simulink model "OfflineSim_V6_nobow"  (R2015a)
settings: Solver=ode3  SolverMode=SingleTasking  StartTime=0.0  StopTime=inf  FixedStep=0.01  RelTol=1e-3
undefined symbols (not defined in the file): BiasOffset, eta_dot_ini, K2, L1, L2, L3
libraries: sldrtlib x1, simulink x1
settings Model: CovMetricSettings=dwe  CovHtmlReporting=off  covSaveCumulativeToWorkspaceVar=off  CovSaveSingleToWorkspaceVar=off  CovExternalEMLEnable=on  Creator=ssp  LastModifiedBy=ssp
settings DataIOCC: LimitDataPoints=off  SaveFormat=Dataset
settings DebuggingCC: SFUnexpectedBacktrackingDiag=error  SFNoUnconditionalDefaultTransitionDiag=error
settings HardwareCC: ProdBitPerPointer=64  ProdLargestAtomicFloat=Float  ProdIntDivRoundTo=Zero  ProdEndianess=LittleEndian  ProdHWDeviceType=Specified
settings ModelReferenceCC: PropagateSignalLabelsOutOfModel=on
settings GRTTargetCC: TargetLangStandard=C99 (ISO)  GeneratePreprocessorConditionals=Use local settings

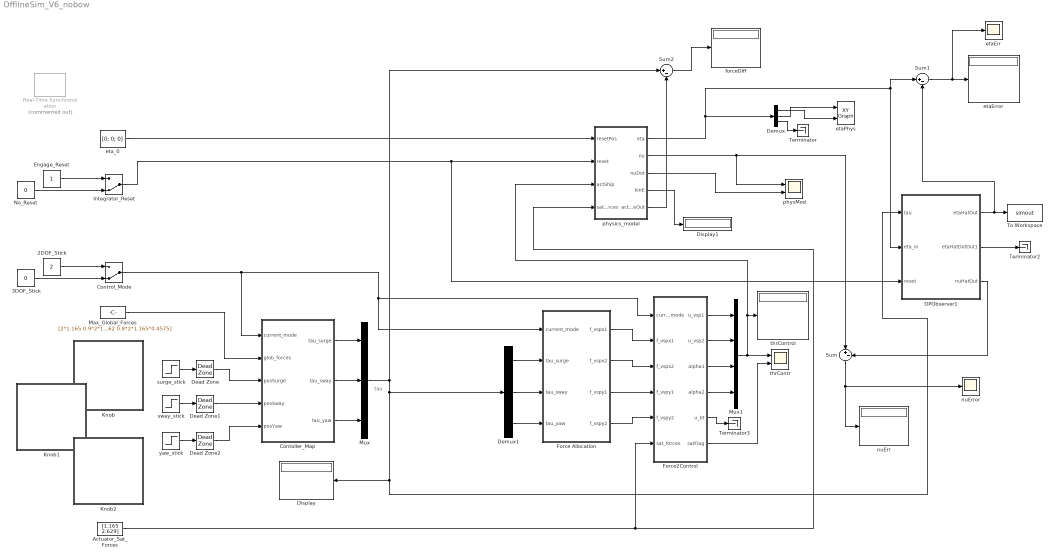
== system OfflineSim_V6_nobow ==
  note: tau
  2DOF_Stick : Constant  Value=2
  3DOF_Stick : Constant  Value=0
  Actuator_Sat_Forces : Constant  Value=[1.165 2.629]
  Contoller_Map : MATLAB Function  TreatAsAtomicUnit=on
      settings: PermitHierarchicalResolution=ParametersOnly
  Control_Mode : ManualSwitch  CurrentSetting=0
  DPObserver1 : Subsystem
  Dead Zone : DeadZone  LowerValue=-0.05  UpperValue=0.05  SaturateOnIntegerOverflow=on
  Dead Zone1 : DeadZone  LowerValue=-0.05  UpperValue=0.05  SaturateOnIntegerOverflow=on
  Dead Zone2 : DeadZone  LowerValue=-0.05  UpperValue=0.05  SaturateOnIntegerOverflow=on
  Demux : Demux  Outputs=3
  Demux1 : Demux  Outputs=3
  Display : Display
  Display1 : Display
  Engage_Reset : Constant
  Force Allocation : MATLAB Function  TreatAsAtomicUnit=on
      settings: PermitHierarchicalResolution=ParametersOnly
  Force2Control : MATLAB Function  TreatAsAtomicUnit=on
      settings: PermitHierarchicalResolution=ParametersOnly
  Integrator_Reset : ManualSwitch  CurrentSetting=0
  Knob : Subsystem  DialogController=hmiCreateDDGDialog  IsWebBlock=on  mask(MathWorksWebBlock){webBlockId=4a71b7a3-6536-403a-8bad-6aeba5635746, webBlockType=continuousknob, ShowInLibBrowser=on, ShowInitialText=on, HMISrcModelName=OfflineSim_V6_nobow}
      mask prompts: webBlockId "WebBlock Id"; webBlockType "WebBlock Type"; HMISrcModelName "Source Model"
      mask help: SimulinkHMI:dialogs:ContinuousKnobDialogDesc
      mask Help: helpview([docroot '/mapfiles/simulink.map'], 'hmi_knob')
      mask Display:
      | if strcmp(get_param(bdroot(gcb),'BlockDiagramType'), 'library')
      |     image([(matlabroot) '/toolbox/simulink/hmi/icons/ContinuousKnob.png']);
      | end
  Knob1 : Subsystem  DialogController=hmiCreateDDGDialog  IsWebBlock=on  mask(MathWorksWebBlock){webBlockId=6469085c-47a6-49a2-9ebc-fb6a8e18618c, webBlockType=continuousknob, ShowInLibBrowser=on, ShowInitialText=on, HMISrcModelName=OfflineSim_V6_nobow}
      mask prompts: webBlockId "WebBlock Id"; webBlockType "WebBlock Type"; HMISrcModelName "Source Model"
      mask help: SimulinkHMI:dialogs:ContinuousKnobDialogDesc
      mask Help: helpview([docroot '/mapfiles/simulink.map'], 'hmi_knob')
      mask Display:
      | if strcmp(get_param(bdroot(gcb),'BlockDiagramType'), 'library')
      |     image([(matlabroot) '/toolbox/simulink/hmi/icons/ContinuousKnob.png']);
      | end
  Knob2 : Subsystem  DialogController=hmiCreateDDGDialog  IsWebBlock=on  mask(MathWorksWebBlock){webBlockId=01ffebd2-c22d-44d7-8fc7-1049d6cabe31, webBlockType=continuousknob, ShowInLibBrowser=on, ShowInitialText=on, HMISrcModelName=OfflineSim_V6_nobow}
      mask prompts: webBlockId "WebBlock Id"; webBlockType "WebBlock Type"; HMISrcModelName "Source Model"
      mask help: SimulinkHMI:dialogs:ContinuousKnobDialogDesc
      mask Help: helpview([docroot '/mapfiles/simulink.map'], 'hmi_knob')
      mask Display:
      | if strcmp(get_param(bdroot(gcb),'BlockDiagramType'), 'library')
      |     image([(matlabroot) '/toolbox/simulink/hmi/icons/ContinuousKnob.png']);
      | end
  Max_Global_Forces : Constant  Value=[2*1.165 0.9*2*1.165*sin(atan(0.062/0.4575)) 0.95*2*1.165*0.062 0.8*2*1.165*0.4575]
  Mux : Mux  Inputs=3
  Mux1 : Mux
  No_Reset : Constant  Value=0
  Real-Time Synchronization : sldrtlib/Real-Time Synchronization  Commented=on  SampleTime=0.1  MaxMissedTicks=10  ShowMissedTicks=off  YieldWhenWaiting=off
  Sum : Sum  Inputs=|+-
  Sum1 : Sum  Inputs=|+-
  Sum2 : Sum  Inputs=|+-
  Terminator : Terminator
  Terminator2 : Terminator
  Terminator3 : Terminator
  To Workspace : ToWorkspace  VariableName=simout  SampleTime=-1
  etaErr : Scope
      settings: TimeRange=50  ShowLegends=on  MaxDataPoints=5000  SaveToWorkspace=off  SaveName=ScopeData2  YMin=-1.00000  YMax=1.00000  SampleTime=-1
  etaError : Display
  etaPhys : simulink/Sinks/XY Graph  xmin=-10  xmax=10  ymin=-10  ymax=10  st=-1
  eta_0 : Constant  Value=[0; 0; 0]
  forceDiff : Display
  nuErr : Display
  nuError : Scope
      settings: TimeRange=50  ShowLegends=on  MaxDataPoints=5000  SaveToWorkspace=off  YMin=-1.00000  YMax=1.00000  SampleTime=-1
  physMod : Scope  NumInputPorts=2
      settings: TimeRange=50  ShowLegends=on  MaxDataPoints=5000  SaveToWorkspace=off  SaveName=ScopeData  YMin=-0.00713~-5  YMax=0.05351~5  SampleTime=-1
  physics_model : Subsystem
  surge_stick : Step  Time=0  After=0  SampleTime=0.01
  sway_stick : Step  Time=0  After=0  SampleTime=0
  thrContr : Scope  NumInputPorts=2
      settings: TimeRange=50  ShowLegends=on  MaxDataPoints=5000  SaveToWorkspace=off  YMin=-0.3927~-5  YMax=3.53429~5  SampleTime=-1
  thrControl : Display
  yaw_stick : Step  Time=0  After=0  SampleTime=0
  wires:
  Engage_Reset/1 -> Integrator_Reset/1
  No_Reset/1 -> Integrator_Reset/2
  Contoller_Map/1(tau_surge) -> Mux/1
  Contoller_Map/2(tau_sway) -> Mux/2
  Contoller_Map/3(tau_yaw) -> Mux/3
  Max_Global_Forces/1 -> Contoller_Map/2(glob_forces)
  2DOF_Stick/1 -> Control_Mode/1
  3DOF_Stick/1 -> Control_Mode/2
  Control_Mode/1 -> Contoller_Map/1(current_mode), Force2Control/1(current_mode), Force Allocation/1(current_mode)
  surge_stick/1 -> Dead Zone/1
  sway_stick/1 -> Dead Zone1/1
  yaw_stick/1 -> Dead Zone2/1
  eta_0/1 -> physics_model/1(resetPos)
  Integrator_Reset/1 -> DPObserver1/3("reset "), physics_model/2(reset)
  Mux/1 -> Sum2/1, Display/1, DPObserver1/1(tau), Demux1/1
  physics_model/1(eta) -> Demux/1, DPObserver1/2(eta_in), Sum1/1
  physics_model/2(nu) -> physMod/1, Sum/1
  Demux/1 -> etaPhys/2
  Demux/2 -> etaPhys/1
  Demux/3 -> Terminator/1
  physics_model/3(nuDot) -> physMod/2
  physics_model/4(kinE) -> Display1/1
  Demux1/1 -> Force Allocation/2(tau_surge)
  Demux1/2 -> Force Allocation/3(tau_sway)
  Demux1/3 -> Force Allocation/4(tau_yaw)
  Force Allocation/1(f_vspx1) -> Force2Control/2(f_vspx1)
  Force Allocation/2(f_vspx2) -> Force2Control/3(f_vspx2)
  Mux1/1 -> thrContr/1, physics_model/3(actShip), thrControl/1
  Force2Control/1(u_vsp1) -> Mux1/1
  Force2Control/2(u_vsp2) -> Mux1/2
  Force2Control/6(satFlag) -> thrContr/2
  Actuator_Sat_Forces/1 -> physics_model/4(satForces), Force2Control/6(sat_forces)
  Dead Zone/1 -> Contoller_Map/3(posSurge)
  Dead Zone1/1 -> Contoller_Map/4(posSway)
  Dead Zone2/1 -> Contoller_Map/5(posYaw)
  DPObserver1/2(etaHatDotOut1) -> Terminator2/1
  DPObserver1/3(nuHatOut) -> Sum/2
  Sum/1 -> nuError/1, nuErr/1
  DPObserver1/1(etaHatOut) -> Sum1/2, To Workspace/1
  Sum1/1 -> etaErr/1, etaError/1
  Force Allocation/3(f_vspy1) -> Force2Control/4(f_vspy1)
  Force Allocation/4(f_vspy2) -> Force2Control/5(f_vspy2)
  Force2Control/5(u_bt) -> Terminator3/1
  Force2Control/3(alpha1) -> Mux1/3
  Force2Control/4(alpha2) -> Mux1/4
  physics_model/5(actForceOut) -> Sum2/2
  Sum2/1 -> forceDiff/1

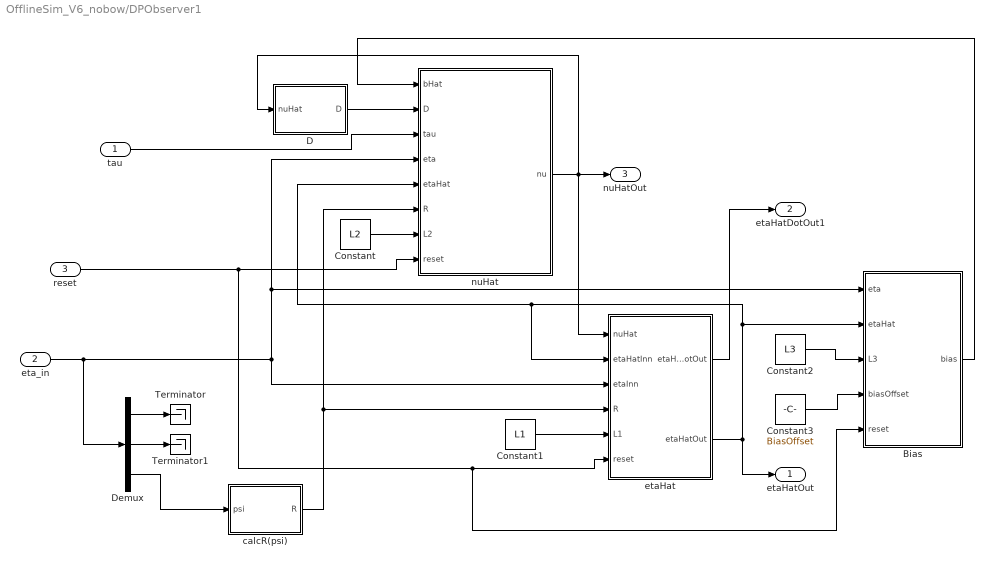
== system OfflineSim_V6_nobow/DPObserver1 ==
  tau : Inport
  eta_in : Inport  Port=2
  "reset " : Inport  Port=3
  Bias : Subsystem
  Constant : Constant  Value=L2
  Constant1 : Constant  Value=L1
  Constant2 : Constant  Value=L3
  Constant3 : Constant  Value=BiasOffset
  D : MATLAB Function  TreatAsAtomicUnit=on
      settings: PermitHierarchicalResolution=ParametersOnly
  Demux : Demux  Outputs=3
  Terminator : Terminator
  Terminator1 : Terminator
  "calcR(psi) " : MATLAB Function  TreatAsAtomicUnit=on
      settings: PermitHierarchicalResolution=ParametersOnly
  etaHat : Subsystem
  nuHat : Subsystem
  etaHatOut : Outport
  etaHatDotOut1 : Outport  Port=2
  nuHatOut : Outport  Port=3
  wires:
  "calcR(psi) "/1(R) -> nuHat/6(R), etaHat/4(R)
  etaHat/2(etaHatOut) -> etaHatOut/1, nuHat/5(etaHat), etaHat/2(etaHatInn), Bias/2(etaHat)
  tau/1 -> nuHat/3(tau)
  etaHat/1(etaHatDotOut) -> etaHatDotOut1/1
  nuHat/1(nu) -> etaHat/1(nuHat), D/1(nuHat), nuHatOut/1
  eta_in/1 -> Demux/1, nuHat/4(eta), Bias/1(eta), etaHat/3(etaInn)
  D/1(D) -> nuHat/2(D)
  Bias/1(bias) -> nuHat/1(bHat)
  Demux/3 -> "calcR(psi) "/1(psi)
  Constant/1 -> nuHat/7(L2)
  Constant2/1 -> Bias/3(L3)
  Constant3/1 -> Bias/4(biasOffset)
  Demux/1 -> Terminator/1
  Demux/2 -> Terminator1/1
  Constant1/1 -> etaHat/5(L1)
  "reset "/1 -> Bias/5(reset), etaHat/6(reset), nuHat/8(reset)

== system OfflineSim_V6_nobow/Knob ==

== system OfflineSim_V6_nobow/Knob1 ==

== system OfflineSim_V6_nobow/Knob2 ==

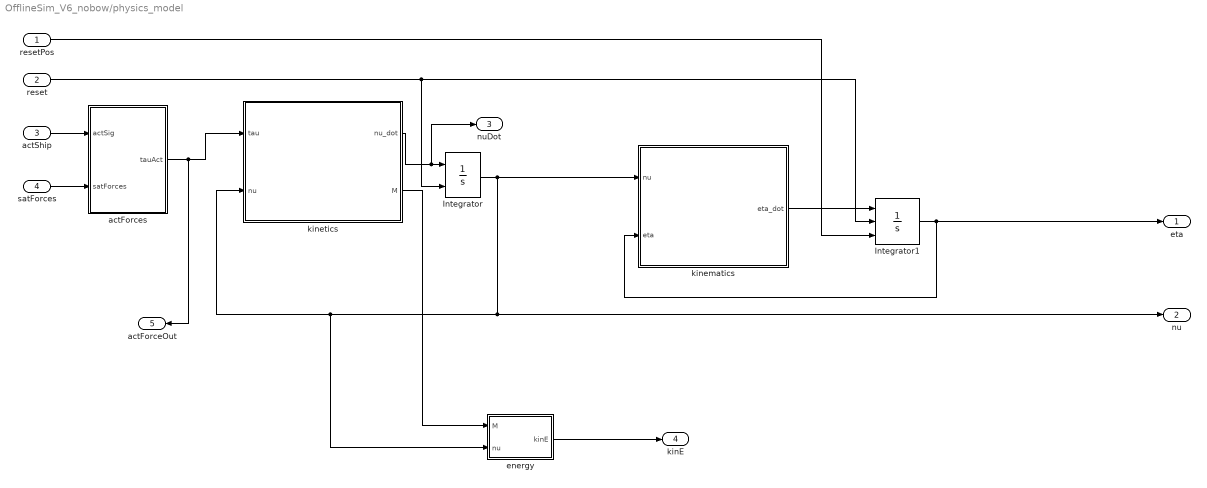
== system OfflineSim_V6_nobow/physics_model ==
  resetPos : Inport
  reset : Inport  Port=2
  actShip : Inport  Port=3
  satForces : Inport  Port=4
  Integrator : Integrator  ExternalReset=rising  InitialCondition=[0 0 0]'
  Integrator1 : Integrator  ExternalReset=rising  InitialConditionSource=external  InitialCondition=[0 0 0]'
  actForces : MATLAB Function  TreatAsAtomicUnit=on
      settings: PermitHierarchicalResolution=ParametersOnly
  energy : MATLAB Function  TreatAsAtomicUnit=on
      settings: PermitHierarchicalResolution=ParametersOnly
  kinematics : MATLAB Function  TreatAsAtomicUnit=on
      settings: PermitHierarchicalResolution=ParametersOnly
  kinetics : MATLAB Function  TreatAsAtomicUnit=on
      settings: PermitHierarchicalResolution=ParametersOnly
  eta : Outport
  nu : Outport  Port=2
  nuDot : Outport  Port=3
  kinE : Outport  Port=4
  actForceOut : Outport  Port=5
  wires:
  kinetics/1(nu_dot) -> nuDot/1, Integrator/1
  Integrator/1 -> nu/1, energy/2(nu), kinetics/2(nu), kinematics/1(nu)
  kinematics/1(eta_dot) -> Integrator1/1
  Integrator1/1 -> eta/1, kinematics/2(eta)
  reset/1 -> Integrator1/2, Integrator/2
  resetPos/1 -> Integrator1/3
  kinetics/2(M) -> energy/1(M)
  energy/1(kinE) -> kinE/1
  actShip/1 -> actForces/1(actSig)
  satForces/1 -> actForces/2(satForces)
  actForces/1(tauAct) -> actForceOut/1, kinetics/1(tau)

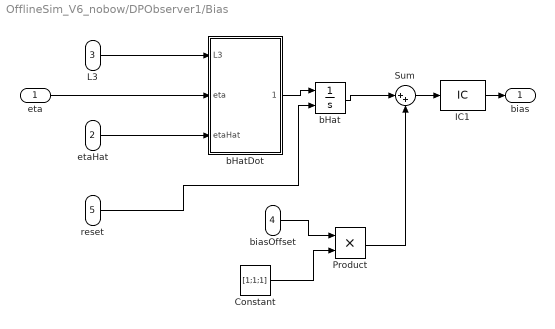
== system OfflineSim_V6_nobow/DPObserver1/Bias ==
  eta : Inport
  etaHat : Inport  Port=2
  L3 : Inport  Port=3
  biasOffset : Inport  Port=4  PortDimensions=1
  reset : Inport  Port=5
  Constant : Constant  Value=[1;1;1]
  IC1 : InitialCondition  Value=[0;0;0]
  Product : Product
  Sum : Sum  Inputs=|++
  bHat : Integrator  ExternalReset=rising
  bHatDot : MATLAB Function  TreatAsAtomicUnit=on
      settings: PermitHierarchicalResolution=ParametersOnly
  bias : Outport
  wires:
  bHatDot/1(bHatDot) -> bHat/1
  eta/1 -> bHatDot/2(eta)
  etaHat/1 -> bHatDot/3(etaHat)
  L3/1 -> bHatDot/1(L3)
  IC1/1 -> bias/1
  Sum/1 -> IC1/1
  biasOffset/1 -> Product/1
  Product/1 -> Sum/2
  Constant/1 -> Product/2
  bHat/1 -> Sum/1
  reset/1 -> bHat/2

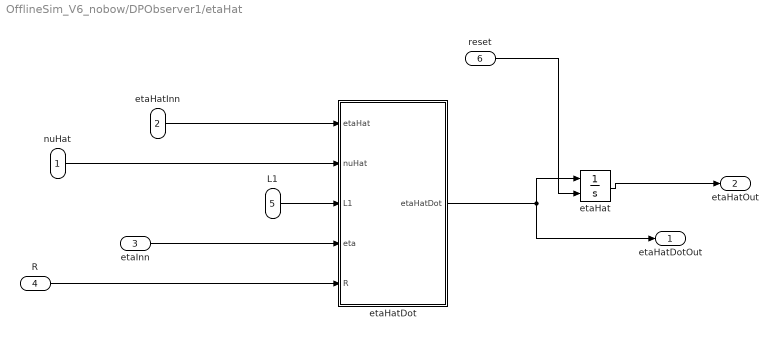
== system OfflineSim_V6_nobow/DPObserver1/etaHat ==
  nuHat : Inport
  etaHatInn : Inport  Port=2
  etaInn : Inport  Port=3
  R : Inport  Port=4
  L1 : Inport  Port=5
  reset : Inport  Port=6
  etaHat : Integrator  ExternalReset=rising  InitialCondition=eta_dot_ini
  etaHatDot : MATLAB Function  TreatAsAtomicUnit=on
      settings: PermitHierarchicalResolution=ParametersOnly
  etaHatDotOut : Outport
  etaHatOut : Outport  Port=2
  wires:
  etaHat/1 -> etaHatOut/1
  etaHatDot/1(etaHatDot) -> etaHat/1, etaHatDotOut/1
  L1/1 -> etaHatDot/3(L1)
  R/1 -> etaHatDot/5(R)
  nuHat/1 -> etaHatDot/2(nuHat)
  etaInn/1 -> etaHatDot/4(eta)
  etaHatInn/1 -> etaHatDot/1(etaHat)
  reset/1 -> etaHat/2

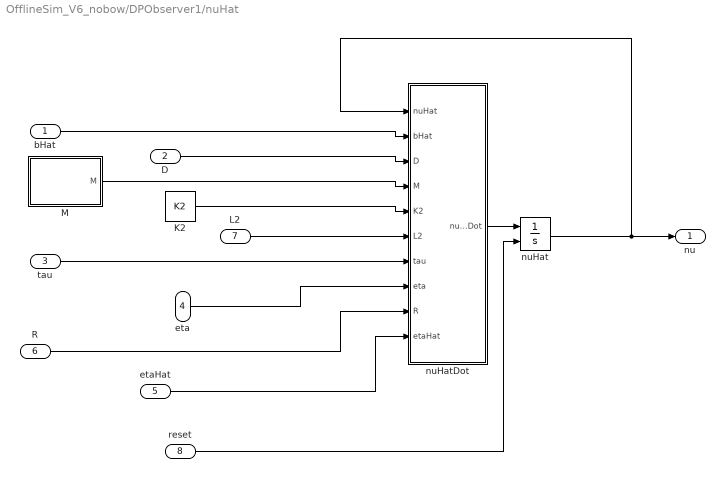
== system OfflineSim_V6_nobow/DPObserver1/nuHat ==
  bHat : Inport
  D : Inport  Port=2
  tau : Inport  Port=3
  eta : Inport  Port=4
  etaHat : Inport  Port=5
  R : Inport  Port=6
  L2 : Inport  Port=7
  reset : Inport  Port=8
  K2 : Constant  Value=K2
  M : MATLAB Function  TreatAsAtomicUnit=on
      settings: PermitHierarchicalResolution=ParametersOnly
  nuHat : Integrator  ExternalReset=rising  InitialCondition=[0;0;0]
  nuHatDot : MATLAB Function  TreatAsAtomicUnit=on
      settings: PermitHierarchicalResolution=ParametersOnly
  nu : Outport
  wires:
  K2/1 -> nuHatDot/5(K2)
  tau/1 -> nuHatDot/7(tau)
  bHat/1 -> nuHatDot/2(bHat)
  M/1(M) -> nuHatDot/4(M)
  nuHat/1 -> nuHatDot/1(nuHat), nu/1
  etaHat/1 -> nuHatDot/10(etaHat)
  R/1 -> nuHatDot/9(R)
  eta/1 -> nuHatDot/8(eta)
  nuHatDot/1(nuHatDot) -> nuHat/1
  D/1 -> nuHatDot/3(D)
  L2/1 -> nuHatDot/6(L2)
  reset/1 -> nuHat/2

== matlab function OfflineSim_V6_nobow/physics_model/kinematics ==
  data: nu input; eta_dot output; eta input
function eta_dot = CSE1_eta_dot(nu,eta)

psi = eta(3);

J = [cos(psi) -sin(psi) 0
     sin(psi) cos(psi)  0
     0        0         1];

eta_dot = J*nu;

== matlab function OfflineSim_V6_nobow/physics_model/kinetics ==
  data: tau input; nu_dot output; nu input; M output
function [nu_dot,M] = CSE1_nu_dot_corr(tau,nu)

u   = nu(1);
v   = nu(2);
r   = nu(3);

tau = [tau(1);tau(2);tau(3)];
%% MATRICES

m    = 14.79;   I_z  =  1.7600;   x_g = 0.0375;       % x_g  =  0.0460; % Table B.1


%% Added mass
X_ud  =     -2.0;											% Table B.1
Y_vd =     -10.0;	
N_vd =    -0.0;                                             % Table B.1 guestimate
Y_rd =      -0.0;	
N_rd =    -1.0;                                             % Table B.1

%% Total mass matrix
m_11 = m-X_ud;
m_22 = m-Y_vd;
m_23 = m*x_g-Y_rd;
m_32 = m*x_g-N_vd;
m_33 = I_z-N_rd;

M    = [m_11 0    0
        0    m_22 m_23
        0    m_32 m_33];
	
%% Damping coefficients
% Comments at the end of the lines indicate the old values used.
X_u		= -0.6555;		X_v		= 0;
X_uu 	= 0.3545;		X_vv	= -2.443;
X_uuu 	= -3.787;		X_vvv	= 0;

Y_v		= -1.33; 			Y_r		= -7.250; % Y_r
Y_vv	= -2.776;			Y_rr	= -3.450; % Y_rr
Y_vvv	= -64.91;			Y_rrr	= 0;
						
Y_rv	= -0.805;			Y_vr	= -0.845; % Y_rv, Y_vr

N_v		= 0;				N_r		= -1.900; % N_r
N_vv	= -0.2088;			N_rr	= -0.750; % N_rr
N_vvv	= 0;				N_rrr	= 0;
N_rv	= 0.130;			N_vr	= 0.080; % N_rv, N_vr

%% Correolis matrix

%from ItsLearning
%  c_13 = -(m-Y_vd)*v-(m*x_g-Y_rd)*r;
%  c_23 = (m-X_ud)*u;
% C    = [0     0     c_13
%         0     0     c_23
%         -c_13 -c_23 0   ];

%From Handbook of Marine Craft Hydr 1st ed pp.120
a1 = X_ud*u;
a2 = Y_vd*v-m*x_g;
C    = [0     0     a2
        0     0    -a1
       -a2    a1    0   ];

%% Assembly of the damping matrix
d_11 = -X_u - X_uu*abs(u) - X_uuu*u^2;
d_22 = -Y_v - Y_vv*abs(v) - Y_vvv*v^2 - Y_rv*abs(r);
d_33 = -N_r - N_rr*abs(r) - N_rrr*r^2 - N_vr*abs(v); % using abs(r)

%d_12 = -X_v - X_vv*abs(v) - X_vvv*v^2;
d_23 = -Y_r - Y_rr*abs(r) - Y_rrr*r^2 - Y_vr*abs(v);
d_32 = -N_v - N_vv*abs(v) - N_vvv*v^2 - N_rv*abs(r);

%From ItsLearning
% D    = [d_11 d_12 0
%         0    d_22 d_23
%         0    d_32 d_33];

%From Feb. 2017 lab manual. Agrees with Handbook of Marine Craft Hydro
D    = [d_11 0    0
        0    d_22 d_23
        0    d_32 d_33];



%% CALCULATION

%nu_dot = M\(tau-(C+D)*nu);
nu_dot = M\(tau-(D)*nu);

== matlab function OfflineSim_V6_nobow/Contoller_Map ==
  data: current_mode input; glob_forces input; posSurge input; posSway input; posYaw input; tau_surge output; tau_sway output; tau_yaw output
function [tau_surge,tau_sway,tau_yaw] = fcn(current_mode,glob_forces,posSurge,posSway,posYaw)

if current_mode==2
    tau_surge=posSurge*glob_forces(1);
    tau_sway=-posYaw*glob_forces(4);
    tau_yaw=0; 
else
    tau_surge=posSurge*glob_forces(1);
    tau_sway=posSway*glob_forces(2);
    tau_yaw=posYaw*glob_forces(3);
end

end

== matlab function OfflineSim_V6_nobow/physics_model/energy ==
  data: M input; kinE output; nu input
function kinE = fcn(M,nu)

kinE=transpose(nu)*M*nu;

== matlab function OfflineSim_V6_nobow/Force Allocation ==
  data: current_mode input; tau_surge input; f_vspx1 output; tau_sway input; tau_yaw input; f_vspx2 output; f_vspy1 output; f_vspy2 output
function [f_vspx1,f_vspx2,f_vspy1,f_vspy2] = fcn(current_mode,tau_surge,tau_sway,tau_yaw)
l_bt=0.3875;
l_vsp=-0.4575;

if current_mode==2
    %2DOF stick control
    f_vspx1=tau_surge/2;
    f_vspx2=f_vspx1;
    f_vspy1=tau_sway/2;
    f_vspy2=f_vspy1;    
else
    %3 DOF stick control, no BT
    f_vspx1_surge=tau_surge/2;
    f_vspx2_surge=f_vspx1_surge;
    
    f_vspy1_sway=tau_sway/2;
    f_vspy2_sway=f_vspy1_sway;
    
    f_vspx1_yaw=0.5*tau_yaw/0.062;
    f_vspx2_yaw=-f_vspx1_yaw;
    
    f_vspx1_sway=f_vspy1_sway*0.4575/0.062;
    f_vspx2_sway=-f_vspx1_sway;
    
    f_vspx1=f_vspx1_surge+f_vspx1_yaw+f_vspx1_sway;
    f_vspx2=f_vspx2_surge+f_vspx2_yaw+f_vspx2_sway;
    f_vspy1=f_vspy1_sway;
    f_vspy2=f_vspy2_sway;
end

%original equations from 30/1/2017
% f_vspx=tau_surge;
% f_vspy=(tau_yaw-tau_sway*l_bt)/(l_vsp-l_bt);
% f_bt=tau_sway-f_vspy;

%tau_yaw = f_vspy*l_vsp+f_bt*l_bt
%tau_sway=f_vspy+f_bt
%solve for f_bt and f_vspy

end

== matlab function OfflineSim_V6_nobow/Force2Control ==
  data: current_mode input; f_vspx1 input; u_vsp1 output; f_vspx2 input; f_vspy1 input; f_vspy2 input; u_vsp2 output; alpha1 output; alpha2 output; u_bt output; sat_forces input; satFlag output
function [u_vsp1,u_vsp2,alpha1,alpha2,u_bt,satFlag] = fcn(current_mode,f_vspx1,f_vspx2,f_vspy1,f_vspy2,sat_forces)

if current_mode==2
    u_vsp1=sqrt(f_vspx1^2+f_vspy1^2)/sat_forces(1);
    u_vsp2=u_vsp1;
    alpha1=atan2(f_vspy1,f_vspx1);
    alpha2=alpha1;
else
    u_vsp1=sqrt(f_vspx1^2+f_vspy1^2)/sat_forces(1);
    u_vsp2=sqrt(f_vspx2^2+f_vspy2^2)/sat_forces(1);
    alpha1=atan2(f_vspy1,f_vspx1);
    alpha2=atan2(f_vspy2,f_vspx2);
end

if abs(u_vsp1) > 1
    sf=1/abs(u_vsp1);
    satFlag=1;
elseif abs(u_vsp2) > 1
    sf=1/abs(u_vsp2);
    satFlag=1;
else
    sf=1;
    satFlag=0;
end

u_vsp1=u_vsp1*sf;
u_vsp2=u_vsp2*sf;
u_bt=0;

end

== matlab function OfflineSim_V6_nobow/physics_model/actForces ==
  data: actSig input; tauAct output; satForces input
function tauAct  = act2Force(actSig,satForces)

t11=actSig(1)*satForces(1)*cos(actSig(3));
t12=actSig(2)*satForces(1)*cos(actSig(4));
t21=actSig(1)*satForces(1)*sin(actSig(3));
t22=actSig(2)*satForces(1)*sin(actSig(4));
t3=(t11-t12)*0.062-(t21+t22)*0.4575;

tauAct=[t11+t12;t21+t22;t3];

== matlab function OfflineSim_V6_nobow/DPObserver1/Bias/bHatDot ==
  data: bHatDot output; L3 input; eta input; etaHat input
function bHatDot = fcn(L3,eta,etaHat)

bHatDot=L3*(eta-etaHat);
%bHatDot=[0;0;0];

end

== matlab function OfflineSim_V6_nobow/DPObserver1/D ==
  data: D output; nuHat input
function D = fcn(nuHat)

u=nuHat(1);     %u=0; 
v=nuHat(2);     %v=0; 
r=nuHat(3);     %r=0;

Xu=-0.6555;
Xuu=0.3545;
Xuuu=-3.787;
Yv=-1.33;
Yvv=-2.776;
Yvvv=-64.91;
Yr=-7.25;
Yrr=-3.45;
Yrrr=0;
Yrv=-0.805;
Yvr=-0.845;
Nv=0;
Nvv=-0.2088;
Nvvv=0;
Nr=-1.9;
Nrr=-0.75;
Nrrr=0;
Nrv=0.13;
Nvr=0.08;

d11=-Xu-Xuu*abs(u)-Xuuu*u^2;
d22=-Yv-Yvv*abs(v)-Yvvv*v^2-Yrv*abs(r);
d23=-Yr-Yvr*abs(v)-Yrr*abs(r)-Yrrr*r^2;
d32=-Nv-Nvv*abs(v)-Nvvv*v^2-Nrv*abs(r);
d33=-Nr-Nvr*abs(v)-Nrr*abs(r)-Nrrr*r^2;

D=[d11 0 0; 0 d22 d23; 0 d32 d33];

end

== matlab function OfflineSim_V6_nobow/DPObserver1/nuHat/M ==
  data: M output
function M = void

m=14.79;
M=[m+2 0 0; 0 m+10 m*0.0375; 0 m*0.0375 1.76+1];

end

== matlab function OfflineSim_V6_nobow/DPObserver1/nuHat/nuHatDot ==
  data: nuHat input; bHat input; D input; M input; K2 input; L2 input; tau input; eta input; R input; etaHat input; nuHatDot output
function nuHatDot = fcn(nuHat,bHat,D,M,K2,L2,tau,eta,R,etaHat)

nuHatDot=inv(M)*(-D*nuHat+transpose(R)*bHat+tau+K2*transpose(R)*L2*(eta-etaHat));

end

== matlab function OfflineSim_V6_nobow/DPObserver1/calcR(psi)  ==
  data: psi input; R output
function R = fcn(psi)

R=[cos(psi) -sin(psi) 0; sin(psi) cos(psi) 0; 0 0 1];

end

== matlab function OfflineSim_V6_nobow/DPObserver1/etaHat/etaHatDot ==
  data: etaHat input; nuHat input; L1 input; eta input; R input; etaHatDot output
function etaHatDot = fcn(etaHat,nuHat,L1,eta,R)

%etaHatDot=zeros(3,1);
etaHatDot=R*nuHat+L1*(eta-etaHat);

end
